simulink model "untitled1"  (R2018a)
settings: Solver=VariableStepAuto  StartTime=0.0  StopTime=10.0  RelTol=1e-3
settings Model: Creator=12969  LastModifiedBy=12969

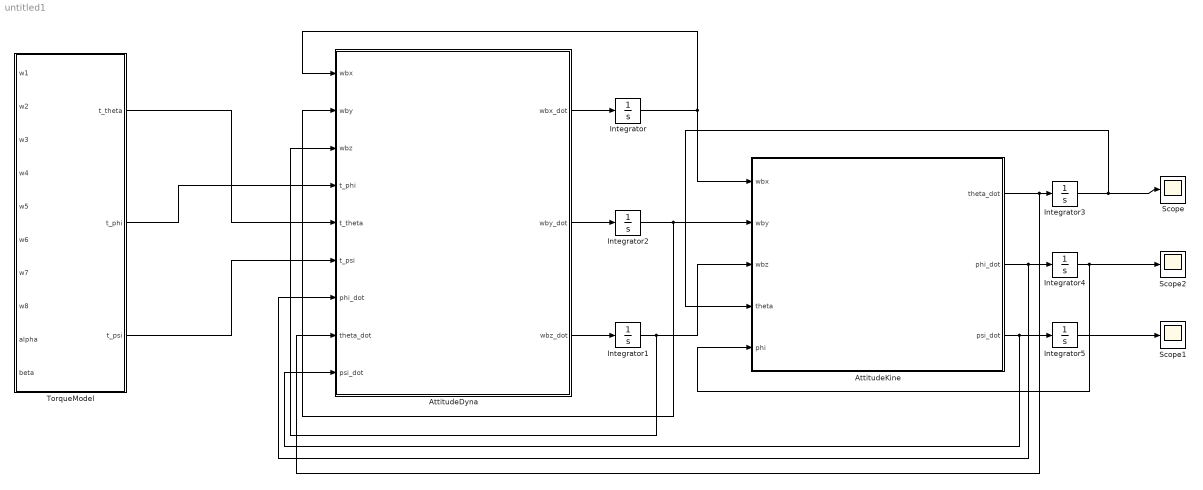
== system untitled1 ==
  AttitudeDyna : MATLAB Function  TreatAsAtomicUnit=on
  AttitudeKine : MATLAB Function  TreatAsAtomicUnit=on
  Integrator{,1..5} (6 alike) : Integrator
  Scope : Scope
  Scope1 : Scope
  Scope2 : Scope
  TorqueModel : MATLAB Function  TreatAsAtomicUnit=on
  wires:
  TorqueModel/1(t_theta) -> AttitudeDyna/5(t_theta)
  TorqueModel/2(t_phi) -> AttitudeDyna/4(t_phi)
  TorqueModel/3(t_psi) -> AttitudeDyna/6(t_psi)
  AttitudeDyna/1(wbx_dot) -> Integrator/1
  AttitudeDyna/2(wby_dot) -> Integrator2/1
  AttitudeDyna/3(wbz_dot) -> Integrator1/1
  Integrator/1 -> AttitudeDyna/1(wbx), AttitudeKine/1(wbx)
  Integrator2/1 -> AttitudeDyna/2(wby), AttitudeKine/2(wby)
  Integrator1/1 -> AttitudeDyna/3(wbz), AttitudeKine/3(wbz)
  AttitudeKine/1(theta_dot) -> AttitudeDyna/8(theta_dot), Integrator3/1
  AttitudeKine/2(phi_dot) -> AttitudeDyna/7(phi_dot), Integrator4/1
  AttitudeKine/3(psi_dot) -> AttitudeDyna/9(psi_dot), Integrator5/1
  Integrator3/1 -> Scope/1, AttitudeKine/4(theta)
  Integrator4/1 -> Scope2/1, AttitudeKine/5(phi)
  Integrator5/1 -> Scope1/1

== matlab function untitled1/AttitudeKine ==
  data: wbx input; theta_dot output; wby input; wbz input; theta input; phi input; phi_dot output; psi_dot output
% wbx,wby,wbz -- 机体坐标系下的无人机角速度
% theta,phi,psi -- 欧拉角
% theta_dot,phi_dot,psi_dot -- 欧拉角角速率
% 将机体坐标系下的角速率转化为世界坐标系下的姿态变换率
function [theta_dot, phi_dot, psi_dot] = AttitudeKine(wbx, wby, wbz, theta, phi)
    theta_dot = wbx + tan(theta)*sin(phi)*wby + tan(theta)*cos(phi)*wbz;
    phi_dot = cos(phi)*wby - sin(phi)*wbz;
    psi_dot = sin(phi)/cos(phi)*wby + cos(phi)/cos(theta)*wbz;
end

== matlab function untitled1/TorqueModel ==
  data: w1 input; t_theta output; w2 input; w3 input; w4 input; w5 input; w6 input; w7 input; w8 input; alpha input; beta input; t_phi output; t_psi output
function [t_theta, t_phi, t_psi] = TorqueModel(w1, w2, w3, w4, w5, w6, w7, w8, alpha, beta)
    l = 330; % 轴距
    u = 1; % 转速与推力的比例系数
    k = 1; % 反扭系数
    t_phi = l*u*(sin(alpha)*w4^2 - sin(beta)*w2^2 + sin(alpha)*w8^2 - sin(beta)*w6^2) + k(cos(alpha)*w4^2 - cos(alpha)*w8^2 + cos(beta)*w2^2 - cos(beta)*w6^2);
    t_theta = l*u*(w1^2 - w3^2 + w5^2 - w7^2);
    t_psi = k(-w1^2 + w5^2 - w3^2 + w7^2 + sin(alpha)*w4^2 - sin(alpha)*w8^2 + sin(beta)*w2^2 - sin(beta)*w6^2);
end

== matlab function untitled1/AttitudeDyna ==
  data: wbx input; wbx_dot output; wby input; wbz input; t_phi input; t_theta input; t_psi input; phi_dot input; theta_dot input; psi_dot input; wby_dot output; wbz_dot output
function [wbx_dot, wby_dot, wbz_dot] = AttitudeDyna(wbx, wby, wbz, t_phi, t_theta, t_psi, phi_dot, theta_dot, psi_dot)
    d = 1000; % 水密度 1000kg/m3
%     c1 = ; % 阻力系数
%     c2 = ;
%     c3 = ;
%     I1 = ; % 转动惯量
%     I2 = ;
%     I3 = ;
    wbx_dot = t_phi/I1 - (I3-I2)*wby*wbz/I1 - d*c1*abs(phi_dot)*wbx/I1;
    wby_dot = t_theta/I2 - (I1-I2)*wbx*wbz/I2 - d*c2*abs(theta_dot)*wby/I2;
    wbz_dot = t_psi/I3 - (I2-I1)*wbx*wbz/I3 - d*c2*abs(psi_dot)*wby/I3;
end
